simulink model "TestCANtransmit"  (R2023b)
settings: Solver=FixedStepAuto  StartTime=0.0  StopTime=inf  RelTol=1e-3  EnableMultiTasking=on
libraries: arduinolib x4, canmsglib x3
settings Model: ExtModeTrigDuration=2  Creator=Pablo  LastModifiedBy=pablo
settings OptimizationCC: EnhancedBackFolding=on  PassReuseOutputArgsAs=Individual arguments  ZeroExternalMemoryAtStartup=off  ZeroInternalMemoryAtStartup=off  MaxStackSize=64  OptimizeBlockOrder=speed  DifferentSizesBufferReuse=on  OptimizationCustomize=off  EfficientTunableParamExpr=on
settings DebuggingCC: ParameterTunabilityLossMsg=error
settings HardwareCC: ProdBitPerPointer=32  ProdBitPerSizeT=32  ProdBitPerPtrDiffT=32  ProdLargestAtomicInteger=Long  ProdLargestAtomicFloat=Double  ProdWordSize=32  ProdHWDeviceType=ARM Compatible->ARM Cortex
settings SFSimCC: MATLABDynamicMemAlloc=off
settings RTWCC: Description=Embedded Coder  SystemTargetFile=ert.tlc  HardwareBoard=Arduino MKR WiFi 1010  TemplateMakefile=ert_default_tmf  Toolchain=Arduino ARM  BuildConfiguration=Faster Runs
settings CodeAppCC: ForceParamTrailComments=on  IgnoreCustomStorageClasses=off  OperatorAnnotations=on  SimulinkDataObjDesc=on  SFDataObjDesc=on  InsertBlockDesc=on
settings ERTTargetCC: SupportContinuousTime=on  SupportVariableSizeSignals=on  ExtMode=on  ExtModeTransport=3  ExtModeStaticAlloc=on  ExtModeAutomaticAllocSize=off  ExtModeStaticAllocSize=8192  ExtModeMexFile=ext_xcp  ExtModeMexArgs=0 5 921600  ExtModeIntrfLevel=Level2 - Open

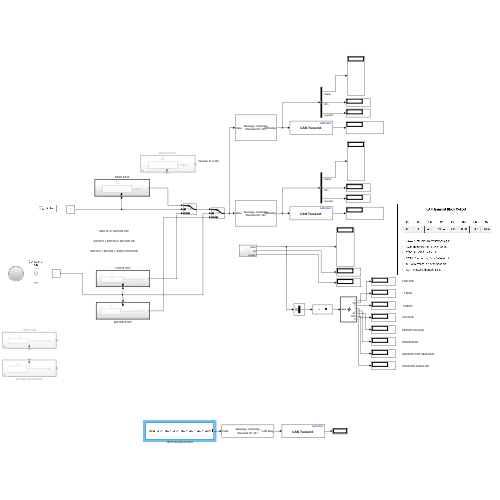
[thumbnail: Simulink's stored preview of the top-level diagram]
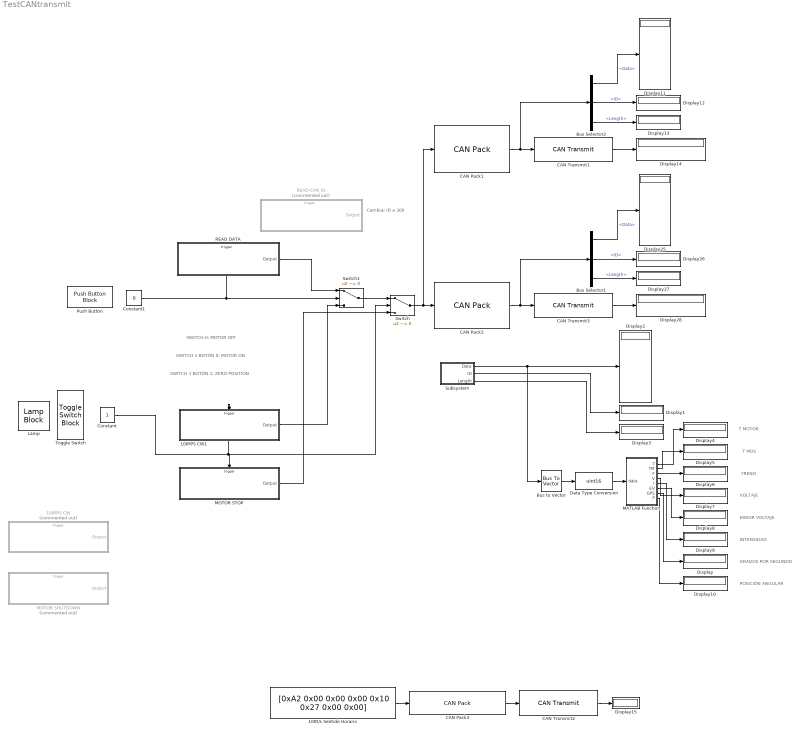
== system TestCANtransmit ==
  note: Cambiar ID a 300
  note: POSICIÓN ANGULAR
  note: GRADOS POR SEGUNDO
  note: INTENSIDAD
  note: ERROR VOLTAJE
  note: VOLTAJE
  note: FRENO
  note: T MOS
  note: T MOTOR
  note: SWITCH 0: MOTOR OFF
  note: SWITCH 1 BOTÓN 1: ZERO POSITION
  note: SWITCH 1 BOTÓN 0: MOTOR ON
  100º/s Sentido Horario : Constant  Value=[0xA2 0x00 0x00 0x00 0x10 0x27 0x00 0x00]  OutDataTypeStr=uint8
  100ºPS CW : Subsystem  Commented=on
  100ºPS CW1 : Subsystem
  Bus Selector1 : BusSelector  OutputSignals=Data,ID,Length
  Bus Selector2 : BusSelector  OutputSignals=Data,ID,Length
  Bus to Vector : BusToVector
  CAN Pack1 : canmsglib/CAN Pack  MsgList=(none)  MsgName=CAN Msg  MsgIDType=Standard (11-bit identifier)  MsgIdentifier=323  MsgLength=8  Remote=off  ApplyMinMax=off  BusOutput=on  SignalInfo={ 'position', '8', '16', 'BE', 'signed', 'Standard', '0', '1', '-95.5', '-95.5', '95.5'; 'velocity', '28', '12', 'BE', 'signed', 'Standard', '0', '1', '-45', '-45', '45'; 'kp', '32', '12', 'BE', 'unsigned', 'Standard', '0', '1', '0', '0', '500'; 'kd', '52', '12', 'BE', 'unsigned', 'Standard', '0', '1', '0', '0', '5'; 'torque', '56', '12', 'BE', 'signed', 'Standard', '0', '1', '-18', '-18', '18' }
      settings: LibrarySourceBlock=embeddedtargetslib/Host Communication/CAN Pack  DataFormat=raw data
  CAN Pack2 : canmsglib/CAN Pack  MsgList=(none)  MsgName=CAN Msg  MsgIDType=Standard (11-bit identifier)  MsgIdentifier=322  MsgLength=8  Remote=off  ApplyMinMax=off  BusOutput=on  SignalInfo={ 'position', '8', '16', 'BE', 'signed', 'Standard', '0', '1', '-95.5', '-95.5', '95.5'; 'velocity', '28', '12', 'BE', 'signed', 'Standard', '0', '1', '-45', '-45', '45'; 'kp', '32', '12', 'BE', 'unsigned', 'Standard', '0', '1', '0', '0', '500'; 'kd', '52', '12', 'BE', 'unsigned', 'Standard', '0', '1', '0', '0', '5'; 'torque', '56', '12', 'BE', 'signed', 'Standard', '0', '1', '-18', '-18', '18' }
      settings: LibrarySourceBlock=embeddedtargetslib/Host Communication/CAN Pack  DataFormat=raw data
  CAN Pack3 : canmsglib/CAN Pack  MsgList=(none)  MsgName=CAN Msg  MsgIDType=Standard (11-bit identifier)  MsgIdentifier=321  MsgLength=8  Remote=off  ApplyMinMax=off  BusOutput=on  SignalInfo={ 'position', '8', '16', 'BE', 'signed', 'Standard', '0', '1', '-95.5', '-95.5', '95.5'; 'velocity', '28', '12', 'BE', 'signed', 'Standard', '0', '1', '-45', '-45', '45'; 'kp', '32', '12', 'BE', 'unsigned', 'Standard', '0', '1', '0', '0', '500'; 'kd', '52', '12', 'BE', 'unsigned', 'Standard', '0', '1', '0', '0', '5'; 'torque', '56', '12', 'BE', 'signed', 'Standard', '0', '1', '-18', '-18', '18' }
      settings: LibrarySourceBlock=embeddedtargetslib/Host Communication/CAN Pack  DataFormat=raw data
  CAN Transmit1 : arduinolib/CAN Transmit  inputDataType=CAN Msg  BlockingMode_=on  BlockTimeout_=1  outputStatus=on  identifierType=Standard (11-bit identifier)  messageId=100  msgLength=8  remoteFrame=off
  CAN Transmit2 : arduinolib/CAN Transmit  inputDataType=CAN Msg  BlockingMode_=on  BlockTimeout_=1  outputStatus=on  identifierType=Standard (11-bit identifier)  messageId=100  msgLength=8  remoteFrame=off
  CAN Transmit3 : arduinolib/CAN Transmit  inputDataType=CAN Msg  BlockingMode_=on  BlockTimeout_=1  outputStatus=on  identifierType=Standard (11-bit identifier)  messageId=100  msgLength=8  remoteFrame=off
  Constant : Constant
  Constant1 : Constant  Value=0
  Data Type Conversion : DataTypeConversion  OutDataTypeStr=uint16  SaturateOnIntegerOverflow=off  RndMeth=Floor
  Display{,1..15,25..28} (20 alike) : Display
      Display11 settings: Format=hex (Stored Integer)
      Display14 settings: Format=binary (Stored Integer)
      Display15 settings: Format=binary (Stored Integer)
      Display2 settings: Format=hex (Stored Integer)
      Display25 settings: Format=hex (Stored Integer)
      Display28 settings: Format=binary (Stored Integer)
  Lamp : LampBlock  LabelPosition=Hide
  MATLAB Function : MATLAB Function  TreatAsAtomicUnit=on
  MOTOR SHUTDOWN : Subsystem  Commented=on
  MOTOR STOP : Subsystem
  Push Button : PushButtonBlock  Icon=AntilockBrakeSystem  OffValue=0.000000
  READ CAN ID : Subsystem  Commented=on
  READ DATA : Subsystem
  Subsystem : Subsystem
  Switch : Switch  Criteria=u2 ~= 0  SaturateOnIntegerOverflow=off  InputSameDT=off
  Switch1 : Switch  Criteria=u2 ~= 0  SaturateOnIntegerOverflow=off  InputSameDT=off
  Toggle Switch : ToggleSwitchBlock
      settings: Values={{'Off', 'On'}, [0 1]}
  wires:
  Switch/1 -> CAN Pack1/1, CAN Pack2/1
  Constant/1 -> 100ºPS CW1/Trigger, MOTOR STOP/Trigger, Switch/2
  Switch1/1 -> Switch/1
  100ºPS CW1/1(Output) -> Switch1/3
  CAN Pack2/1 -> CAN Transmit3/1, Bus Selector1/1
  Bus Selector1/2 -> Display26/1  "<ID>"
  Bus Selector1/1 -> Display25/1  "<Data>"
  Bus Selector1/3 -> Display27/1  "<Length>"
  CAN Transmit3/1 -> Display28/1
  Subsystem/1(Data) -> Display2/1, Bus to Vector/1
  Subsystem/2(ID) -> Display1/1
  Subsystem/3(Length) -> Display3/1
  Constant1/1 -> READ DATA/Trigger, Switch1/2
  Bus to Vector/1 -> Data Type Conversion/1
  MATLAB Function/1(T) -> Display4/1
  MATLAB Function/2(TM) -> Display5/1
  MATLAB Function/3(F) -> Display6/1
  MATLAB Function/4(V) -> Display7/1
  MATLAB Function/6(EV) -> Display8/1
  Data Type Conversion/1 -> MATLAB Function/1(data)
  MATLAB Function/5(I) -> Display9/1
  MATLAB Function/7(GPS) -> Display/1
  MATLAB Function/8(P) -> Display10/1
  READ DATA/1(Output) -> Switch1/1
  CAN Transmit1/1 -> Display14/1
  Bus Selector2/2 -> Display12/1  "<ID>"
  Bus Selector2/1 -> Display11/1  "<Data>"
  CAN Pack1/1 -> CAN Transmit1/1, Bus Selector2/1
  Bus Selector2/3 -> Display13/1  "<Length>"
  MOTOR STOP/1(Output) -> Switch/3
  100º/s Sentido Horario/1 -> CAN Pack3/1
  CAN Pack3/1 -> CAN Transmit2/1
  CAN Transmit2/1 -> Display15/1

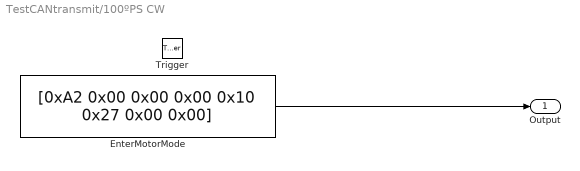
== system TestCANtransmit/100ºPS CW ==
  Trigger : TriggerPort  VariantControl=(inherit)  PortDimensions=1
  EnterMotorMode : Constant  Value=[0xA2 0x00 0x00 0x00 0x10 0x27 0x00 0x00]  OutDataTypeStr=uint8
  Output : Outport
  wires:
  EnterMotorMode/1 -> Output/1

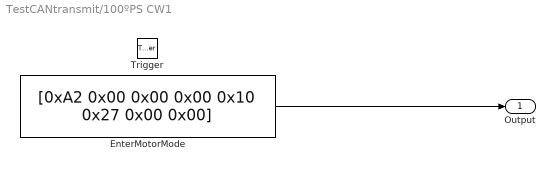
== system TestCANtransmit/100ºPS CW1 ==
  Trigger : TriggerPort  VariantControl=(inherit)  PortDimensions=1
  EnterMotorMode : Constant  Value=[0xA2 0x00 0x00 0x00 0x10 0x27 0x00 0x00]  OutDataTypeStr=uint8
  Output : Outport
  wires:
  EnterMotorMode/1 -> Output/1

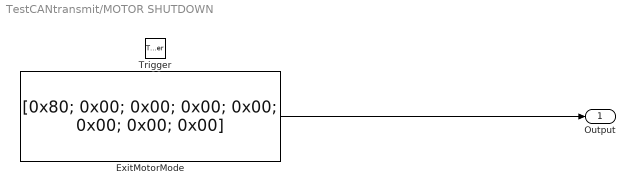
== system TestCANtransmit/MOTOR SHUTDOWN ==
  Trigger : TriggerPort  TriggerType=falling  VariantControl=(inherit)  PortDimensions=1
  ExitMotorMode : Constant  Value=|  OutDataTypeStr=uint8
      | [0x80; 0x00; 0x00; 0x00; 0x00;
      | 0x00;
      | 0x00;
      | 0x00]
  Output : Outport
  wires:
  ExitMotorMode/1 -> Output/1

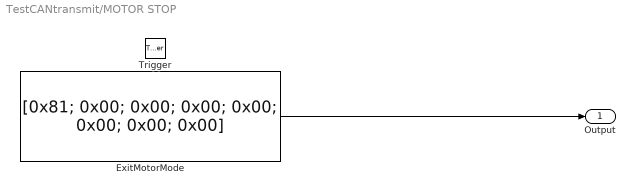
== system TestCANtransmit/MOTOR STOP ==
  Trigger : TriggerPort  TriggerType=falling  VariantControl=(inherit)  PortDimensions=1
  ExitMotorMode : Constant  Value=|  OutDataTypeStr=uint8
      | [0x81; 0x00; 0x00; 0x00; 0x00;
      | 0x00;
      | 0x00;
      | 0x00]
  Output : Outport
  wires:
  ExitMotorMode/1 -> Output/1

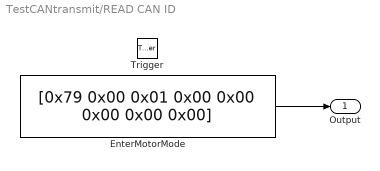
== system TestCANtransmit/READ CAN ID ==
  Trigger : TriggerPort  VariantControl=(inherit)  PortDimensions=1
  EnterMotorMode : Constant  Value=[0x79 0x00 0x01 0x00 0x00 0x00 0x00 0x00]  OutDataTypeStr=uint8
  Output : Outport
  wires:
  EnterMotorMode/1 -> Output/1

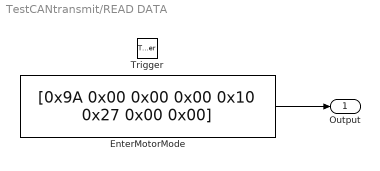
== system TestCANtransmit/READ DATA ==
  Trigger : TriggerPort  VariantControl=(inherit)  PortDimensions=1
  EnterMotorMode : Constant  Value=[0x9A 0x00 0x00 0x00 0x10 0x27 0x00 0x00]  OutDataTypeStr=uint8
  Output : Outport
  wires:
  EnterMotorMode/1 -> Output/1

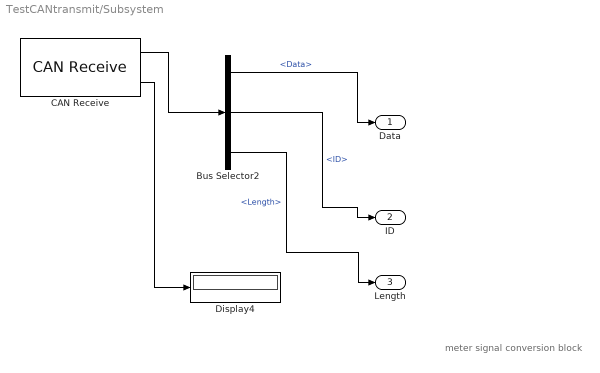
== system TestCANtransmit/Subsystem ==
  note: meter signal conversion block
  Bus Selector2 : BusSelector  OutputSignals=Data,ID,Length
  CAN Receive : arduinolib/CAN Receive  outputDataType=CAN Msg  identifierType=Standard (11-bit identifier)  messageId=100  msgLength=8  SampleTime=0.1  outputError=off  outputRemote=off
  Display4 : Display
  Data : Outport
  ID : Outport  Port=2
  Length : Outport  Port=3
  wires:
  Bus Selector2/1 -> Data/1  "<Data>"
  CAN Receive/2 -> Display4/1
  Bus Selector2/2 -> ID/1  "<ID>"
  Bus Selector2/3 -> Length/1  "<Length>"
  CAN Receive/1 -> Bus Selector2/1

== matlab function TestCANtransmit/MATLAB Function ==
  data: data input; T output; TM output; F output; V output; I output; EV output; GPS output; P output
function [T,TM,F,V,I,EV,GPS,P] = fcn(data)
T=uint8(0);
TM=uint8(0);
F=boolean(0);
V=double(0);
I=double(0);
EV=double(0);
GPS=uint32(0);
P=uint16(0);
data1=data(1);
data2=data(2);
data3=data(3);
data4=data(4);

data5=data(5);
data6=double(data(6));
data7=data(7);
data8=data(8);
switch data1
    case 0x9A %READ DATA
    T = uint8(data2); %T MOTOR
    TM = uint8(data3); %T TUBO MOS
    F = boolean(data4); %FRENO
    V = 0.1*double(256*data6 + data5); %VOLTAJE
    EV = 0.1*double(256*data8 + data7); %ERROR VOLTAJE

    case 0xA2 %100 GPS CW
    T = uint8(data2); %T MOTOR
    I = 0.01*double(256*data4 + data3); %INTENSIDAD
    GPS = uint32(256*data6 + data5); %GRADOS POR SEGUNDO
    P = uint16(256*data8 + data7); %POSICIÓN ANGULAR
end
end
